simulink model "model2"  (R2020b)
settings: Solver=VariableStepAuto  StartTime=0.0  StopTime=300  RelTol=1e-3
undefined symbols (not defined in the file): k, T, tau
settings Model: Creator=48576  LastModifiedBy=48576

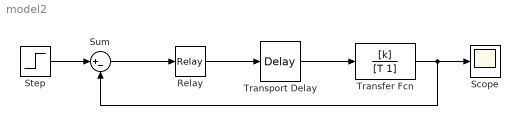
== system model2 ==
  Relay : Relay  OnSwitchValue=0  OffSwitchValue=0  OnOutputValue=5  OffOutputValue=1
  Scope : Scope
  Step : Step  After=2.5  SampleTime=0
  Sum : Sum  Inputs=|+-
  Transfer Fcn : TransferFcn  Numerator=[k]  Denominator=[T 1]
  Transport Delay : TransportDelay  DelayTime=tau  PadeOrder=10
  wires:
  Step/1 -> Sum/1
  Sum/1 -> Relay/1
  Relay/1 -> Transport Delay/1
  Transport Delay/1 -> Transfer Fcn/1
  Transfer Fcn/1 -> Sum/2, Scope/1
